simulink model "NewModuleTry_cs"  (Simulink 8.4)
settings: Solver=ode5  SolverMode=SingleTasking  StartTime=0.0  StopTime=inf  FixedStep=1/100  RelTol=1e-3
PreLoadFcn:
  | mbxruntime.callbacks.PreLoadFcn(bdroot);
PostLoadFcn:
  | mbxruntime.callbacks.PostLoadFcn(bdroot);
InitFcn:
  | mbxruntime.callbacks.InitFcn(bdroot);
StartFcn:
  | mbxruntime.callbacks.StartFcn(bdroot);
StopFcn:
  | mbxruntime.callbacks.StopFcn(bdroot);
undefined symbols (not defined in the file or in its folder): dfreq, gray, InitImageOutputDir, Rec, SDTV, strel
libraries: simulink x41, PreScanSimulinkLibrary x15, visiontextngfix x15, simulink_extras x12, visionconversions x3, PreScanUsefulBlocks x3, visionsinks x2, visionstatistics x1, visionmorphops x1, visionanalysis x1, simulink_need_slupdate x1
(part 2 of 7)

== system NewModuleTry_cs/BMW_Z3_1/DISABLED ==
  SELF_BMW_Z3_1 : Inport  Tag=inport/SelfPort  OutDataTypeStr=Bus: PRESCAN_SELFSENSORDATA  PortDimensions=1  SampleTime=1/100  BusOutputAsStruct=on
  TIS_1 : Inport  Tag=inport/TIS  Port=2  OutDataTypeStr=Bus: PRESCAN_SCANNERSENSOR_MESSAGE  PortDimensions=1  SampleTime=1/25  BusOutputAsStruct=on
  V2X_Rx243_Generic_Receiver : Inport  Tag=inport/plugin/sfun_V2X_Generic_Receiver  Port=3  BusOutputAsStruct=on
  GND1 : Subsystem
  GND2 : Ground
  TRM1 : Terminator
  TRM2 : Terminator
  TRM3 : Terminator
  STATE_BMW_Z3_1_bus : Outport  Tag=outport/StatePort  OutDataTypeStr=Bus: PRESCAN_STATEACTUATORDATA  PortDimensions=1  SampleTime=1/100
  V2X_Tx243_Generic_Transmitter : Outport  Tag=outport/plugin/sfun_V2X_Generic_Transmitter  Port=2
  wires:
  SELF_BMW_Z3_1/1 -> TRM1/1
  TIS_1/1 -> TRM2/1
  V2X_Rx243_Generic_Receiver/1 -> TRM3/1
  GND1/1(bus) -> STATE_BMW_Z3_1_bus/1
  GND2/1 -> V2X_Tx243_Generic_Transmitter/1

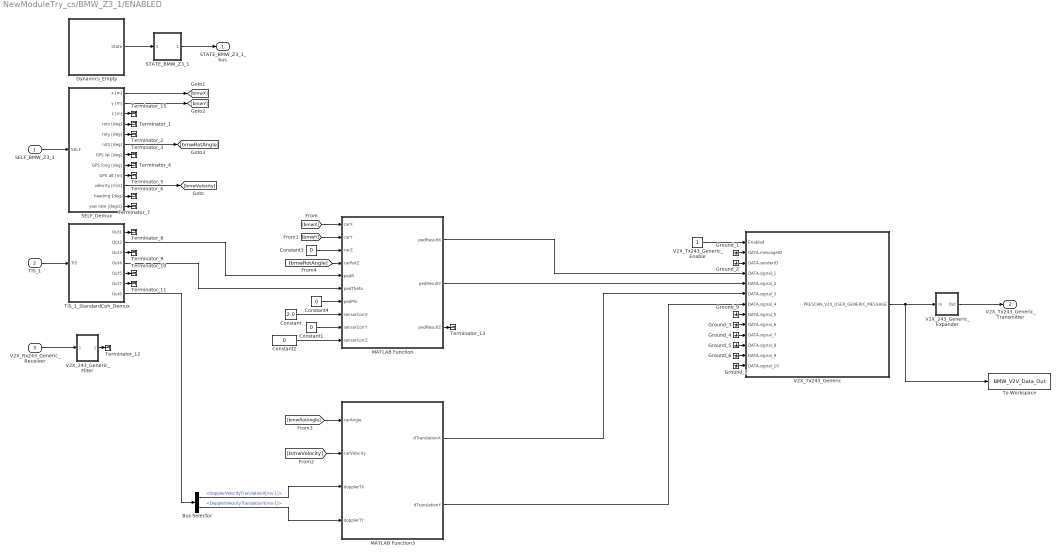
== system NewModuleTry_cs/BMW_Z3_1/ENABLED ==
  SELF_BMW_Z3_1 : Inport  Tag=inport/SelfPort  OutDataTypeStr=Bus: PRESCAN_SELFSENSORDATA  PortDimensions=1  SampleTime=1/100  BusOutputAsStruct=on
  TIS_1 : Inport  Tag=inport/TIS  Port=2  OutDataTypeStr=Bus: PRESCAN_SCANNERSENSOR_MESSAGE  PortDimensions=1  SampleTime=1/25  BusOutputAsStruct=on
  V2X_Rx243_Generic_Receiver : Inport  Tag=inport/plugin/sfun_V2X_Generic_Receiver  Port=3  BusOutputAsStruct=on
  Bus Selector : BusSelector  OutputSignals=DopplerVelocityTranslationX[ms-1],DopplerVelocityTranslationY[ms-1]
  Constant : Constant  Value=2.0
  Constant{1..4} (4 alike) : Constant  Value=0
  Dynamics_Empty : Subsystem  Tag=Dynamics_Empty
      mask Help: eval('openHelp(202)')
      mask Display: port_label('output', 1, 'State');text(0,0,' Empty\n')
  Ground_{1..7,9} (8 alike) : Ground
  MATLAB Function : MATLAB Function  TreatAsAtomicUnit=on
  MATLAB Function3 : MATLAB Function  TreatAsAtomicUnit=on
  SELF_Demux : Subsystem  Tag=demux/SelfPort  mask(PreScan Demux Block:){}
      mask help:
      | The SELF port shows (state) information of the actor itself. The outputs are position in the experiment's axis system and the GPS coordinates, and the object's absolute velocity and compass heading.
      |
      | For more information, please click Help.
      settings: DeleteFcn=PreScanBlockDeleteFcn;
      mask Help: eval('openHelp(462)')
      mask Display:
      | port_label('output',1,'x [m]')
      | port_label('output',2,'y [m]')
      | port_label('output',3,'z [m]','texmode','on')
      | port_label('output',4,'Rotx [deg]','texmode','on')
      | port_label('output',5,'Roty [deg]','texmode','on')
      | port_label('output',6,'Rotz [deg]','texmode','on')
      | port_label('output',7,'GPS lat [deg]','texmode','on')
      | port_label('output',8,'GPS long [deg]','texmode','on')
      | port_label('output',9,'GPS alt [m]','texmode','on')
      | port_label('output',10,'Velocity [m/s]')
      | port_label('output',11,'Heading [deg]')
      | port_label('output',12,'Yaw rate [deg/s]')
  STATE_BMW_Z3_1 : Subsystem  Tag=mux/StatePort  Priority=0  LoadFcn=load PrescanStateActuatorData  mask(PreScan Sink Block: State){x0=126.56578063964844, y0=141.80066680908203, z0=0.4784, Roll0=0, Pitch0=0, Yaw0=270, TimeStep=1/100}
      mask prompts: x0 "Ini x-position VEHICLE wrt GLOBAL axis system [m]"; y0 "Ini y-position VEHICLE wrt GLOBAL axis system [m]"; z0 "Ini z-position VEHICLE wrt GLOBAL axis system [m]"; Roll0 "Ini roll-angle BODY wrt VEHICLE axis system [deg]"; Pitch0 "Ini pitch-angle BODY wrt VEHICLE axis system [deg]"; Yaw0 "Ini yaw-angle VEHICLE wrt GLOBAL axis system [deg]"; TimeStep "Auto-Assigned: Upload Period [s]"
      mask help:
      | The Actor State contains a vector signal of size (9x1), containing the following signals:
      |
      | -  Position                  (x,y,z)                                     [m]
      | -  Velocity                  (vx,vy,vz)                               [m/s]
      | -  Angles                    (Roll, Pitch, Yaw)                   [rad]
      |
      | The Actor state is defined in the global axis system.
      | The state is superponed on the Initial position defined in the GUI.
      |
      | For more information, please click Help.
      settings: DeleteFcn=PreScanBlockDeleteFcn;
      mask Help: eval('openHelp(222)')
      mask Display: image(imread('State.png'))
  TIS_1_StandardCoh_Demux : Subsystem  Tag=demux/TIS/StandardCoh  TreatAsAtomicUnit=on  mask(PreScan Demux Block: TIS){MAXMESSAGES=1}
      mask prompts: MAXMESSAGES "Number of Objects"
      mask Help: eval('openHelp(449)')
      mask Display:
      | port_label('input',1,'TIS')
      | port_label('output',1,'Beam ID [-]')
      | port_label('output',2,'Range [m]')
      | port_label('output',3,'DopplerVelocity [m/s]')
      | port_label('output',4,'{\theta} [deg]','texmode','on')
      | port_label('output',5,'{\phi} [deg]','texmode','on')
      | port_label('output',6,'Target ID [-]','texmode','on')
      | port_label('output',7,'TIS Data','texmode','on')
  Terminator_{1..13,15} (14 alike) : Terminator
  To Workspace : ToWorkspace  VariableName=BMW_V2V_Data_Out  SaveFormat=Timeseries  SampleTime=-1
  V2X_243_Generic_Expander : Subsystem  LoadFcn=addpath .\V2XPlugin; V2Xbusses;
  V2X_243_Generic_Filter : Subsystem
      mask Display: disp('[1]');
  V2X_Tx243_Generic : Subsystem
  V2X_Tx243_Generic_Enable : Constant  OutDataTypeStr=Inherit: Inherit via back propagation
  STATE_BMW_Z3_1_bus : Outport  Tag=outport/StatePort  OutDataTypeStr=Bus: PRESCAN_STATEACTUATORDATA  PortDimensions=1  SampleTime=1/100
  V2X_Tx243_Generic_Transmitter : Outport  Tag=outport/plugin/sfun_V2X_Generic_Transmitter  Port=2
  wires:
  TIS_1_StandardCoh_Demux/2(Out2) -> MATLAB Function/5(pedR)
  TIS_1_StandardCoh_Demux/4(Out4) -> MATLAB Function/6(pedTheta)
  Constant/1 -> MATLAB Function/8(sensorCorrX)
  Constant1/1 -> MATLAB Function/9(sensorCorrY)
  Constant2/1 -> MATLAB Function/10(sensorCorrZ)
  Constant3/1 -> MATLAB Function/3(carZ)
  Constant4/1 -> MATLAB Function/7(pedPhi)
  SELF_Demux/3(z [m]) -> Terminator_15/1
  MATLAB Function/1(pedResultX) -> V2X_Tx243_Generic/4(DATA.signal_1)
  MATLAB Function/2(pedResultY) -> V2X_Tx243_Generic/5(DATA.signal_2)
  TIS_1_StandardCoh_Demux/7(Out6) -> Bus Selector/1
  Bus Selector/1 -> MATLAB Function3/3(dopplerTX)  "<DopplerVelocityTranslationX[ms-1]>"
  Bus Selector/2 -> MATLAB Function3/4(dopplerTY)  "<DopplerVelocityTranslationY[ms-1]>"
  SELF_Demux/10(velocity [m/s]) -> [bmwVelocity]
  SELF_Demux/1(x [m]) -> [bmwX]
  SELF_Demux/2(y [m]) -> [bmwY]
  [bmwX] -> MATLAB Function/1(carX)
  [bmwY] -> MATLAB Function/2(carY)
  SELF_Demux/6(rotz [deg]) -> [bmwRotAngle]
  [bmwVelocity] -> MATLAB Function3/2(carVelocity)
  [bmwRotAngle] -> MATLAB Function3/1(carAngle)
  MATLAB Function3/1(dTranslationX) -> V2X_Tx243_Generic/6(DATA.signal_3)
  MATLAB Function3/2(dTranslationY) -> V2X_Tx243_Generic/7(DATA.signal_4)
  [bmwRotAngle] -> MATLAB Function/4(carRotZ)
  Ground_9/1 -> V2X_Tx243_Generic/8(DATA.signal_5)
  MATLAB Function/3(pedResultZ) -> Terminator_13/1
  V2X_Tx243_Generic/1(PRESCAN_V2X_USER_GENERIC_MESSAGE) -> To Workspace/1, V2X_243_Generic_Expander/1(In)
  STATE_BMW_Z3_1/1(StateBus) -> STATE_BMW_Z3_1_bus/1
  SELF_BMW_Z3_1/1 -> SELF_Demux/1(SELF)
  TIS_1/1 -> TIS_1_StandardCoh_Demux/1(TIS)
  Dynamics_Empty/1(State) -> STATE_BMW_Z3_1/1(State)
  V2X_Tx243_Generic_Enable/1 -> V2X_Tx243_Generic/1(Enabled)
  V2X_243_Generic_Expander/1(Out) -> V2X_Tx243_Generic_Transmitter/1
  V2X_Rx243_Generic_Receiver/1 -> V2X_243_Generic_Filter/1(Filter_In)
  SELF_Demux/4(rotx [deg]) -> Terminator_1/1
  SELF_Demux/5(roty [deg]) -> Terminator_2/1
  SELF_Demux/7(GPS lat [deg]) -> Terminator_3/1
  SELF_Demux/8(GPS long [deg]) -> Terminator_4/1
  SELF_Demux/9(GPS alt [m]) -> Terminator_5/1
  SELF_Demux/11(heading [deg]) -> Terminator_6/1
  SELF_Demux/12(yaw rate [deg/s]) -> Terminator_7/1
  TIS_1_StandardCoh_Demux/1(Out1) -> Terminator_8/1
  TIS_1_StandardCoh_Demux/3(Out3) -> Terminator_9/1
  TIS_1_StandardCoh_Demux/5(Out5) -> Terminator_10/1
  TIS_1_StandardCoh_Demux/6(Out7) -> Terminator_11/1
  V2X_243_Generic_Filter/1(Filter_Out) -> Terminator_12/1
  Ground_1/1 -> V2X_Tx243_Generic/2(DATA.messageID)
  Ground_2/1 -> V2X_Tx243_Generic/3(DATA.senderID)
  Ground_3/1 -> V2X_Tx243_Generic/9(DATA.signal_6)
  Ground_4/1 -> V2X_Tx243_Generic/10(DATA.signal_7)
  Ground_5/1 -> V2X_Tx243_Generic/11(DATA.signal_8)
  Ground_6/1 -> V2X_Tx243_Generic/12(DATA.signal_9)
  Ground_7/1 -> V2X_Tx243_Generic/13(DATA.signal_10)

== system NewModuleTry_cs/CameraSensor_1/DISABLED ==
  GND1 : Ground
  CameraSensor_1 : Outport  Tag=outport/Camera/CameraSensor  OutDataTypeStr=uint8  SampleTime=1/50
  wires:
  GND1/1 -> CameraSensor_1/1

== system NewModuleTry_cs/CameraSensor_1/ENABLED ==
  Sensor : S-Function  FunctionName=sfun_Camera  Parameters=sensorID, dataWidth, dataHeight, channelsPerImage, numberOfImages, timestep  EnableBusSupport=off  mask(PreScan Source Block: Camera Sensor){sensorID=69, dataWidth=375, dataHeight=500, channelsPerImage=1, numberOfImages=1, timestep=1/50}
      mask prompts: sensorID "Sensor ID"; dataWidth "Data width"; dataHeight "Data Height"; channelsPerImage "Channels per image"; numberOfImages "Number of images"; timestep "MATLAB timestep:"
      mask help: The Camera Sensor provides a color or monochrome image.
      mask Help: eval('openHelp(457)')
      mask Display: image(imread('CameraSensor.png'))
  CameraSensor_1 : Outport  Tag=outport/Camera/CameraSensor  OutDataTypeStr=uint8  SampleTime=1/50
  wires:
  Sensor/1 -> CameraSensor_1/1

== system NewModuleTry_cs/CollisionDetection/DISABLED ==
  GND1 : Subsystem
  CollisionDetection : Outport  Tag=outport/CollisionDetection  OutDataTypeStr=Bus: PRESCAN_COLLISIONDETECTION_MESSAGE  PortDimensions=1  SampleTime=1/100
  wires:
  GND1/1(bus) -> CollisionDetection/1

== system NewModuleTry_cs/CollisionDetection/ENABLED ==
  Sensor : S-Function  FunctionName=sfun_CollisionDetection  Parameters=detectableCollisions, timestep  EnableBusSupport=off  mask(PreScan Source Block: CollisionDetection){detectableCollisions=1, timestep=1/100}
      mask prompts: detectableCollisions "Max detectable collisions:"; timestep "MATLAB timestep:"
      mask help: Collision Detection can be used to detect collisions between PreScan components. For Collision Detection the actual component shape is taken into account, so it is not a bounding box approach.
      mask Help: eval('openHelp(811)')
      mask Display: image(imread('crash.jpg'))
  CollisionDetection : Outport  Tag=outport/CollisionDetection  OutDataTypeStr=Bus: PRESCAN_COLLISIONDETECTION_MESSAGE  PortDimensions=1  SampleTime=1/100
  wires:
  Sensor/1 -> CollisionDetection/1

== system NewModuleTry_cs/Male_RegularAni_1/DISABLED ==
  SELF_Male_RegularAni_1 : Inport  Tag=inport/SelfPort  OutDataTypeStr=Bus: PRESCAN_SELFSENSORDATA  PortDimensions=1  SampleTime=1/100  BusOutputAsStruct=on
  GND1 : Subsystem
  GND2 : Subsystem
  TRM1 : Terminator
  STATE_Male_RegularAni_1_bus : Outport  Tag=outport/StatePort  OutDataTypeStr=Bus: PRESCAN_STATEACTUATORDATA  PortDimensions=1  SampleTime=1/100
  ANIM_Male_RegularAni_1 : Outport  Tag=outport/AnimationOutport  Port=2  OutDataTypeStr=Bus: PRESCAN_ANIMACTUATORDATA  PortDimensions=1  SampleTime=1/100
  wires:
  SELF_Male_RegularAni_1/1 -> TRM1/1
  GND1/1(bus) -> STATE_Male_RegularAni_1_bus/1
  GND2/1(bus) -> ANIM_Male_RegularAni_1/1

== system NewModuleTry_cs/Male_RegularAni_1/ENABLED ==
  SELF_Male_RegularAni_1 : Inport  Tag=inport/SelfPort  OutDataTypeStr=Bus: PRESCAN_SELFSENSORDATA  PortDimensions=1  SampleTime=1/100  BusOutputAsStruct=on
  Animation : Subsystem  Tag=RunningHumanAnimation  mask(Prescan Conversion Block: Running Human Animation){MWS=1.95, WalkingScale=1.0, RunningScale=1.0, TimeStep=1/100}
      mask prompts: MWS "Maximum Walking Speed [m/s], above which the animation will switch to running mode."; WalkingScale "Walking mode scaling factor to sync the animation frames to the displacement."; RunningScale "Running mode scaling factor to sync the animation frames to the displacement."; TimeStep "Auto-Assigned: Upload Period [s]"
      mask help: The Running Human Animation block converts the State signal of a human into signals to properly control the animation.
      mask Help: eval('openHelp(239)');
      mask Display: image(imread('HumanAnimated.jpg'))
  SELF_Demux : Subsystem  Tag=demux/SelfPort  mask(PreScan Demux Block:){}
      mask help:
      | The SELF port shows (state) information of the actor itself. The outputs are position in the experiment's axis system and the GPS coordinates, and the object's absolute velocity and compass heading.
      |
      | For more information, please click Help.
      settings: DeleteFcn=PreScanBlockDeleteFcn;
      mask Help: eval('openHelp(462)')
      mask Display:
      | port_label('output',1,'x [m]')
      | port_label('output',2,'y [m]')
      | port_label('output',3,'z [m]','texmode','on')
      | port_label('output',4,'Rotx [deg]','texmode','on')
      | port_label('output',5,'Roty [deg]','texmode','on')
      | port_label('output',6,'Rotz [deg]','texmode','on')
      | port_label('output',7,'GPS lat [deg]','texmode','on')
      | port_label('output',8,'GPS long [deg]','texmode','on')
      | port_label('output',9,'GPS alt [m]','texmode','on')
      | port_label('output',10,'Velocity [m/s]')
      | port_label('output',11,'Heading [deg]')
      | port_label('output',12,'Yaw rate [deg/s]')
  STATE_Male_RegularAni_1 : Subsystem  Tag=mux/StatePort  Priority=0  LoadFcn=load PrescanStateActuatorData  mask(PreScan Sink Block: State){x0=122.28665161132812, y0=124.52811431884766, z0=0, Roll0=0, Pitch0=0, Yaw0=53.000965224957312, TimeStep=1/100}
      mask prompts: x0 "Ini x-position VEHICLE wrt GLOBAL axis system [m]"; y0 "Ini y-position VEHICLE wrt GLOBAL axis system [m]"; z0 "Ini z-position VEHICLE wrt GLOBAL axis system [m]"; Roll0 "Ini roll-angle BODY wrt VEHICLE axis system [deg]"; Pitch0 "Ini pitch-angle BODY wrt VEHICLE axis system [deg]"; Yaw0 "Ini yaw-angle VEHICLE wrt GLOBAL axis system [deg]"; TimeStep "Auto-Assigned: Upload Period [s]"
      mask help:
      | The Actor State contains a vector signal of size (9x1), containing the following signals:
      |
      | -  Position                  (x,y,z)                                     [m]
      | -  Velocity                  (vx,vy,vz)                               [m/s]
      | -  Angles                    (Roll, Pitch, Yaw)                   [rad]
      |
      | The Actor state is defined in the global axis system.
      | The state is superponed on the Initial position defined in the GUI.
      |
      | For more information, please click Help.
      settings: DeleteFcn=PreScanBlockDeleteFcn;
      mask Help: eval('openHelp(222)')
      mask Display: image(imread('State.png'))
  Terminator_{1..12} (12 alike) : Terminator
  Trajectories : Subsystem  Tag=Trajectories  mask(PreScan Source Block: Trajectories){}
      mask help:
      | The Trajectory block contains the trajectories defined in the PreScan Experiment Editor. The output of the trajectory block is the (vehicle) State.
      |
      | For more information, please click Help.
      settings: DeleteFcn=PreScanBlockDeleteFcn;
      mask Help: eval('openHelp(312)')
      mask Display: image(imread('Trajectory.png'));
  STATE_Male_RegularAni_1_bus : Outport  Tag=outport/StatePort  OutDataTypeStr=Bus: PRESCAN_STATEACTUATORDATA  PortDimensions=1  SampleTime=1/100
  ANIM_Male_RegularAni_1 : Outport  Tag=outport/AnimationOutport  Port=2  OutDataTypeStr=Bus: PRESCAN_ANIMACTUATORDATA  PortDimensions=1  SampleTime=1/100
  wires:
  STATE_Male_RegularAni_1/1(StateBus) -> STATE_Male_RegularAni_1_bus/1, Animation/1(In1)
  Animation/1(Out1) -> ANIM_Male_RegularAni_1/1
  SELF_Male_RegularAni_1/1 -> SELF_Demux/1(SELF)
  Trajectories/1(State) -> STATE_Male_RegularAni_1/1(State)
  SELF_Demux/1(x [m]) -> Terminator_1/1
  SELF_Demux/2(y [m]) -> Terminator_2/1
  SELF_Demux/3(z [m]) -> Terminator_3/1
  SELF_Demux/4(rotx [deg]) -> Terminator_4/1
  SELF_Demux/5(roty [deg]) -> Terminator_5/1
  SELF_Demux/6(rotz [deg]) -> Terminator_6/1
  SELF_Demux/7(GPS lat [deg]) -> Terminator_7/1
  SELF_Demux/8(GPS long [deg]) -> Terminator_8/1
  SELF_Demux/9(GPS alt [m]) -> Terminator_9/1
  SELF_Demux/10(velocity [m/s]) -> Terminator_10/1
  SELF_Demux/11(heading [deg]) -> Terminator_11/1
  SELF_Demux/12(yaw rate [deg/s]) -> Terminator_12/1

== system NewModuleTry_cs/SELF_Audi_A8_1/DISABLED ==
  GND1 : Subsystem
  SELF_Audi_A8_1 : Outport  Tag=outport/SelfPort  OutDataTypeStr=Bus: PRESCAN_SELFSENSORDATA  PortDimensions=1  SampleTime=1/100
  wires:
  GND1/1(bus) -> SELF_Audi_A8_1/1

== system NewModuleTry_cs/SELF_Audi_A8_1/ENABLED ==
  Sensor : S-Function  FunctionName=sfun_SelfSensor  Parameters=UniqueID, TimeStep  EnableBusSupport=off  mask(PreScan Source Block: SELF){UniqueID=58, TimeStep=1/100}
      mask prompts: UniqueID "Auto-Assigned: Unique ID"; TimeStep "Auto-Assigned: Upload Period [s]"
      mask help:
      | The SELF port shows (state) information of the actor itself. The outputs are position in the experiment's axis system and the GPS coordinates, and the object's absolute velocity and compass heading.
      |
      | For more information, please click Help.
      mask Help: eval('openHelp(462)')
      mask Display: image(imread('GPS.png'))
  SELF_Audi_A8_1 : Outport  Tag=outport/SelfPort  OutDataTypeStr=Bus: PRESCAN_SELFSENSORDATA  PortDimensions=1  SampleTime=1/100
  wires:
  Sensor/1 -> SELF_Audi_A8_1/1

== system NewModuleTry_cs/SELF_BMW_Z3_1/DISABLED ==
  GND1 : Subsystem
  SELF_BMW_Z3_1 : Outport  Tag=outport/SelfPort  OutDataTypeStr=Bus: PRESCAN_SELFSENSORDATA  PortDimensions=1  SampleTime=1/100
  wires:
  GND1/1(bus) -> SELF_BMW_Z3_1/1

== system NewModuleTry_cs/SELF_BMW_Z3_1/ENABLED ==
  Sensor : S-Function  FunctionName=sfun_SelfSensor  Parameters=UniqueID, TimeStep  EnableBusSupport=off  mask(PreScan Source Block: SELF){UniqueID=59, TimeStep=1/100}
      mask prompts: UniqueID "Auto-Assigned: Unique ID"; TimeStep "Auto-Assigned: Upload Period [s]"
      mask help:
      | The SELF port shows (state) information of the actor itself. The outputs are position in the experiment's axis system and the GPS coordinates, and the object's absolute velocity and compass heading.
      |
      | For more information, please click Help.
      mask Help: eval('openHelp(462)')
      mask Display: image(imread('GPS.png'))
  SELF_BMW_Z3_1 : Outport  Tag=outport/SelfPort  OutDataTypeStr=Bus: PRESCAN_SELFSENSORDATA  PortDimensions=1  SampleTime=1/100
  wires:
  Sensor/1 -> SELF_BMW_Z3_1/1

== system NewModuleTry_cs/SELF_Male_RegularAni_1/DISABLED ==
  GND1 : Subsystem
  SELF_Male_RegularAni_1 : Outport  Tag=outport/SelfPort  OutDataTypeStr=Bus: PRESCAN_SELFSENSORDATA  PortDimensions=1  SampleTime=1/100
  wires:
  GND1/1(bus) -> SELF_Male_RegularAni_1/1

== system NewModuleTry_cs/SELF_Male_RegularAni_1/ENABLED ==
  Sensor : S-Function  FunctionName=sfun_SelfSensor  Parameters=UniqueID, TimeStep  EnableBusSupport=off  mask(PreScan Source Block: SELF){UniqueID=60, TimeStep=1/100}
      mask prompts: UniqueID "Auto-Assigned: Unique ID"; TimeStep "Auto-Assigned: Upload Period [s]"
      mask help:
      | The SELF port shows (state) information of the actor itself. The outputs are position in the experiment's axis system and the GPS coordinates, and the object's absolute velocity and compass heading.
      |
      | For more information, please click Help.
      mask Help: eval('openHelp(462)')
      mask Display: image(imread('GPS.png'))
  SELF_Male_RegularAni_1 : Outport  Tag=outport/SelfPort  OutDataTypeStr=Bus: PRESCAN_SELFSENSORDATA  PortDimensions=1  SampleTime=1/100
  wires:
  Sensor/1 -> SELF_Male_RegularAni_1/1

== system NewModuleTry_cs/STATE_Audi_A8_1_bus/DISABLED ==
  STATE_Audi_A8_1_bus : Inport  Tag=inport/StatePort  OutDataTypeStr=Bus: PRESCAN_STATEACTUATORDATA  PortDimensions=1  SampleTime=1/100  BusOutputAsStruct=on
  TRM1 : Terminator
  wires:
  STATE_Audi_A8_1_bus/1 -> TRM1/1

== system NewModuleTry_cs/STATE_Audi_A8_1_bus/ENABLED ==
  STATE_Audi_A8_1_bus : Inport  Tag=inport/StatePort  OutDataTypeStr=Bus: PRESCAN_STATEACTUATORDATA  PortDimensions=1  SampleTime=1/100  BusOutputAsStruct=on
  Actuator : S-Function  FunctionName=sfun_StateActuator  Parameters=UniqueID, TimeStep  EnableBusSupport=off  mask(PreScan Sink Block: State){UniqueID=58, TimeStep=1/100}
      mask prompts: UniqueID "Auto-Assigned: Unique ID"; TimeStep "Auto-Assigned: Upload Period [s]"
      mask help:
      | The Actor State contains a vector signal of size (9x1), containing the following signals:
      |
      | -  Position    	(x,y,z)             	[m]
      | -  Velocity    	(vx,vy,vz)         	[m/s]
      | -  Angles       	(Roll, Pitch, Yaw)	[rad]
      |
      | The Actor state is defined in the global axis system.
      | The state is superponed on the Initial position defined in the GUI.
      |
      | For more information, please click Help.
      mask Help: eval('openHelp(222)')
      mask Display: image(imread('State.png'))
  wires:
  STATE_Audi_A8_1_bus/1 -> Actuator/1

== system NewModuleTry_cs/STATE_BMW_Z3_1_bus/DISABLED ==
  STATE_BMW_Z3_1_bus : Inport  Tag=inport/StatePort  OutDataTypeStr=Bus: PRESCAN_STATEACTUATORDATA  PortDimensions=1  SampleTime=1/100  BusOutputAsStruct=on
  TRM1 : Terminator
  wires:
  STATE_BMW_Z3_1_bus/1 -> TRM1/1

== system NewModuleTry_cs/STATE_BMW_Z3_1_bus/ENABLED ==
  STATE_BMW_Z3_1_bus : Inport  Tag=inport/StatePort  OutDataTypeStr=Bus: PRESCAN_STATEACTUATORDATA  PortDimensions=1  SampleTime=1/100  BusOutputAsStruct=on
  Actuator : S-Function  FunctionName=sfun_StateActuator  Parameters=UniqueID, TimeStep  EnableBusSupport=off  mask(PreScan Sink Block: State){UniqueID=59, TimeStep=1/100}
      mask prompts: UniqueID "Auto-Assigned: Unique ID"; TimeStep "Auto-Assigned: Upload Period [s]"
      mask help:
      | The Actor State contains a vector signal of size (9x1), containing the following signals:
      |
      | -  Position    	(x,y,z)             	[m]
      | -  Velocity    	(vx,vy,vz)         	[m/s]
      | -  Angles       	(Roll, Pitch, Yaw)	[rad]
      |
      | The Actor state is defined in the global axis system.
      | The state is superponed on the Initial position defined in the GUI.
      |
      | For more information, please click Help.
      mask Help: eval('openHelp(222)')
      mask Display: image(imread('State.png'))
  wires:
  STATE_BMW_Z3_1_bus/1 -> Actuator/1

== system NewModuleTry_cs/STATE_Male_RegularAni_1_bus/DISABLED ==
  STATE_Male_RegularAni_1_bus : Inport  Tag=inport/StatePort  OutDataTypeStr=Bus: PRESCAN_STATEACTUATORDATA  PortDimensions=1  SampleTime=1/100  BusOutputAsStruct=on
  TRM1 : Terminator
  wires:
  STATE_Male_RegularAni_1_bus/1 -> TRM1/1

== system NewModuleTry_cs/STATE_Male_RegularAni_1_bus/ENABLED ==
  STATE_Male_RegularAni_1_bus : Inport  Tag=inport/StatePort  OutDataTypeStr=Bus: PRESCAN_STATEACTUATORDATA  PortDimensions=1  SampleTime=1/100  BusOutputAsStruct=on
  Actuator : S-Function  FunctionName=sfun_StateActuator  Parameters=UniqueID, TimeStep  EnableBusSupport=off  mask(PreScan Sink Block: State){UniqueID=60, TimeStep=1/100}
      mask prompts: UniqueID "Auto-Assigned: Unique ID"; TimeStep "Auto-Assigned: Upload Period [s]"
      mask help:
      | The Actor State contains a vector signal of size (9x1), containing the following signals:
      |
      | -  Position    	(x,y,z)             	[m]
      | -  Velocity    	(vx,vy,vz)         	[m/s]
      | -  Angles       	(Roll, Pitch, Yaw)	[rad]
      |
      | The Actor state is defined in the global axis system.
      | The state is superponed on the Initial position defined in the GUI.
      |
      | For more information, please click Help.
      mask Help: eval('openHelp(222)')
      mask Display: image(imread('State.png'))
  wires:
  STATE_Male_RegularAni_1_bus/1 -> Actuator/1

== system NewModuleTry_cs/TIS_1/DISABLED ==
  GND1 : Subsystem
  TIS_1 : Outport  Tag=outport/TIS  OutDataTypeStr=Bus: PRESCAN_SCANNERSENSOR_MESSAGE  PortDimensions=1  SampleTime=1/25
  wires:
  GND1/1(bus) -> TIS_1/1

== system NewModuleTry_cs/TIS_1/ENABLED ==
  Sensor : S-Function  FunctionName=sfun_TIS  Parameters=sensorID, detectableObjects, timestep  EnableBusSupport=off  mask(PreScan Source Block: Technology Independent Sensor (TIS)){sensorID=68, detectableObjects=1, timestep=1/25}
      mask prompts: sensorID "Sensor ID"; detectableObjects "Max detectable objects:"; timestep "MATLAB timestep:"
      mask help:
      | The Technology Independent Sensor (TIS) provides a sensor with all sensor-related influence factors (like noise, drift and accuracy) without being technology specific (like radar and lidar). The TIS detects the closest point on the geometry of an object.
      |
      | For more information, please click Help.
      mask Help: eval('openHelp(449)')
      mask Display: image(imread('TIS.png'))
  TIS_1 : Outport  Tag=outport/TIS  OutDataTypeStr=Bus: PRESCAN_SCANNERSENSOR_MESSAGE  PortDimensions=1  SampleTime=1/25
  wires:
  Sensor/1 -> TIS_1/1

== system NewModuleTry_cs/TIS_2/DISABLED ==
  GND1 : Subsystem
  TIS_2 : Outport  Tag=outport/TIS  OutDataTypeStr=Bus: PRESCAN_SCANNERSENSOR_MESSAGE  PortDimensions=1  SampleTime=1/25
  wires:
  GND1/1(bus) -> TIS_2/1

== system NewModuleTry_cs/TIS_2/ENABLED ==
  Sensor : S-Function  FunctionName=sfun_TIS  Parameters=sensorID, detectableObjects, timestep  EnableBusSupport=off  mask(PreScan Source Block: Technology Independent Sensor (TIS)){sensorID=192, detectableObjects=1, timestep=1/25}
      mask prompts: sensorID "Sensor ID"; detectableObjects "Max detectable objects:"; timestep "MATLAB timestep:"
      mask help:
      | The Technology Independent Sensor (TIS) provides a sensor with all sensor-related influence factors (like noise, drift and accuracy) without being technology specific (like radar and lidar). The TIS detects the closest point on the geometry of an object.
      |
      | For more information, please click Help.
      mask Help: eval('openHelp(449)')
      mask Display: image(imread('TIS.png'))
  TIS_2 : Outport  Tag=outport/TIS  OutDataTypeStr=Bus: PRESCAN_SCANNERSENSOR_MESSAGE  PortDimensions=1  SampleTime=1/25
  wires:
  Sensor/1 -> TIS_2/1

== system NewModuleTry_cs/V2X_Rx243_Generic_Receiver/DISABLED ==
  GND1 : Ground
  V2X_Rx243_Generic_Receiver : Outport  Tag=outport/plugin/sfun_V2X_Generic_Receiver
  wires:
  GND1/1 -> V2X_Rx243_Generic_Receiver/1

== system NewModuleTry_cs/V2X_Rx243_Generic_Receiver/ENABLED ==
  Sensor : S-Function  LoadFcn=load('Generic.mat');  FunctionName=sfun_V2X_Generic_Receiver  Parameters=sensorID, parentID, maxMessages, timestep  EnableBusSupport=off  mask(V2X Generic Receiver Block){sensorID=243, parentID=59, maxMessages=1, timestep=1/100}
      mask prompts: sensorID "Receiver ID"; parentID "Parent ID"; maxMessages "Maximum number of messages"; timestep "MATLAB timestep:"
      mask help: V2X Block receiving a Generic message
      mask Display: image(imread('V2XR_grayscale.png'))
  V2X_Rx243_Generic_Receiver : Outport  Tag=outport/plugin/sfun_V2X_Generic_Receiver
  wires:
  Sensor/1 -> V2X_Rx243_Generic_Receiver/1

== system NewModuleTry_cs/V2X_Rx244_Generic_Receiver/DISABLED ==
  GND1 : Ground
  V2X_Rx244_Generic_Receiver : Outport  Tag=outport/plugin/sfun_V2X_Generic_Receiver
  wires:
  GND1/1 -> V2X_Rx244_Generic_Receiver/1

== system NewModuleTry_cs/V2X_Rx244_Generic_Receiver/ENABLED ==
  Sensor : S-Function  LoadFcn=load('Generic.mat');  FunctionName=sfun_V2X_Generic_Receiver  Parameters=sensorID, parentID, maxMessages, timestep  EnableBusSupport=off  mask(V2X Generic Receiver Block){sensorID=244, parentID=58, maxMessages=1, timestep=1/100}
      mask prompts: sensorID "Receiver ID"; parentID "Parent ID"; maxMessages "Maximum number of messages"; timestep "MATLAB timestep:"
      mask help: V2X Block receiving a Generic message
      mask Display: image(imread('V2XR_grayscale.png'))
  V2X_Rx244_Generic_Receiver : Outport  Tag=outport/plugin/sfun_V2X_Generic_Receiver
  wires:
  Sensor/1 -> V2X_Rx244_Generic_Receiver/1

== system NewModuleTry_cs/V2X_Tx243_Generic_Transmitter/DISABLED ==
  V2X_Tx243_Generic_Transmitter : Inport  Tag=inport/plugin/sfun_V2X_Generic_Transmitter  BusOutputAsStruct=on
  TRM1 : Terminator
  wires:
  V2X_Tx243_Generic_Transmitter/1 -> TRM1/1

== system NewModuleTry_cs/V2X_Tx243_Generic_Transmitter/ENABLED ==
  V2X_Tx243_Generic_Transmitter : Inport  Tag=inport/plugin/sfun_V2X_Generic_Transmitter  BusOutputAsStruct=on
  Actuator : S-Function  LoadFcn=load('Generic.mat');  FunctionName=sfun_V2X_Generic_Transmitter  Parameters=sensorID, parentID, timestep  EnableBusSupport=off  mask(V2X Generic Transmitter Block){sensorID=243, parentID=59, timestep=1/100}
      mask prompts: sensorID "Transmitter ID"; parentID "Parent ID"; timestep "MATLAB timestep:"
      mask help: V2X Block transmitting a Generic message
      mask Display: image(imread('V2XT_grayscale.png'))
  wires:
  V2X_Tx243_Generic_Transmitter/1 -> Actuator/1

== system NewModuleTry_cs/V2X_Tx244_Generic_Transmitter/DISABLED ==
  V2X_Tx244_Generic_Transmitter : Inport  Tag=inport/plugin/sfun_V2X_Generic_Transmitter  BusOutputAsStruct=on
  TRM1 : Terminator
  wires:
  V2X_Tx244_Generic_Transmitter/1 -> TRM1/1

== system NewModuleTry_cs/V2X_Tx244_Generic_Transmitter/ENABLED ==
  V2X_Tx244_Generic_Transmitter : Inport  Tag=inport/plugin/sfun_V2X_Generic_Transmitter  BusOutputAsStruct=on
  Actuator : S-Function  LoadFcn=load('Generic.mat');  FunctionName=sfun_V2X_Generic_Transmitter  Parameters=sensorID, parentID, timestep  EnableBusSupport=off  mask(V2X Generic Transmitter Block){sensorID=244, parentID=58, timestep=1/100}
      mask prompts: sensorID "Transmitter ID"; parentID "Parent ID"; timestep "MATLAB timestep:"
      mask help: V2X Block transmitting a Generic message
      mask Display: image(imread('V2XT_grayscale.png'))
  wires:
  V2X_Tx244_Generic_Transmitter/1 -> Actuator/1

== system NewModuleTry_cs/Audi_A8_1/DISABLED/GND1 ==
  GND_AccelerationX : Constant  Value=0
  GND_AccelerationY : Constant  Value=0
  GND_AccelerationZ : Constant  Value=0
  GND_AngularVelocityPitch : Constant  Value=0
  GND_AngularVelocityRoll : Constant  Value=0
  GND_AngularVelocityYaw : Constant  Value=0
  GND_OrientationPitch : Constant  Value=0
  GND_OrientationRoll : Constant  Value=0
  GND_OrientationYaw : Constant  Value=0
  GND_PositionX : Constant  Value=0
  GND_PositionY : Constant  Value=0
  GND_PositionZ : Constant  Value=0
  GND_VelocityX : Constant  Value=0
  GND_VelocityY : Constant  Value=0
  GND_VelocityZ : Constant  Value=0
  buscreator : BusCreator  Inputs=15  OutDataTypeStr=Bus: PRESCAN_STATEACTUATORDATA  NonVirtualBus=on
  bus : Outport  OutDataTypeStr=Bus: PRESCAN_STATEACTUATORDATA
  wires:
  GND_PositionX/1 -> buscreator/1  "PositionX"
  GND_PositionY/1 -> buscreator/2  "PositionY"
  GND_PositionZ/1 -> buscreator/3  "PositionZ"
  GND_VelocityX/1 -> buscreator/4  "VelocityX"
  GND_VelocityY/1 -> buscreator/5  "VelocityY"
  GND_VelocityZ/1 -> buscreator/6  "VelocityZ"
  GND_AccelerationX/1 -> buscreator/7  "AccelerationX"
  GND_AccelerationY/1 -> buscreator/8  "AccelerationY"
  GND_AccelerationZ/1 -> buscreator/9  "AccelerationZ"
  GND_OrientationRoll/1 -> buscreator/10  "OrientationRoll"
  GND_OrientationPitch/1 -> buscreator/11  "OrientationPitch"
  GND_OrientationYaw/1 -> buscreator/12  "OrientationYaw"
  GND_AngularVelocityRoll/1 -> buscreator/13  "AngularVelocityRoll"
  GND_AngularVelocityPitch/1 -> buscreator/14  "AngularVelocityPitch"
  GND_AngularVelocityYaw/1 -> buscreator/15  "AngularVelocityYaw"
  buscreator/1 -> bus/1

== system NewModuleTry_cs/Audi_A8_1/ENABLED/CameraSensor_1_MM_Demux ==
  note: This block exists for legacy compatibility only
  In1 : Inport
  I : Outport
  wires:
  In1/1 -> I/1

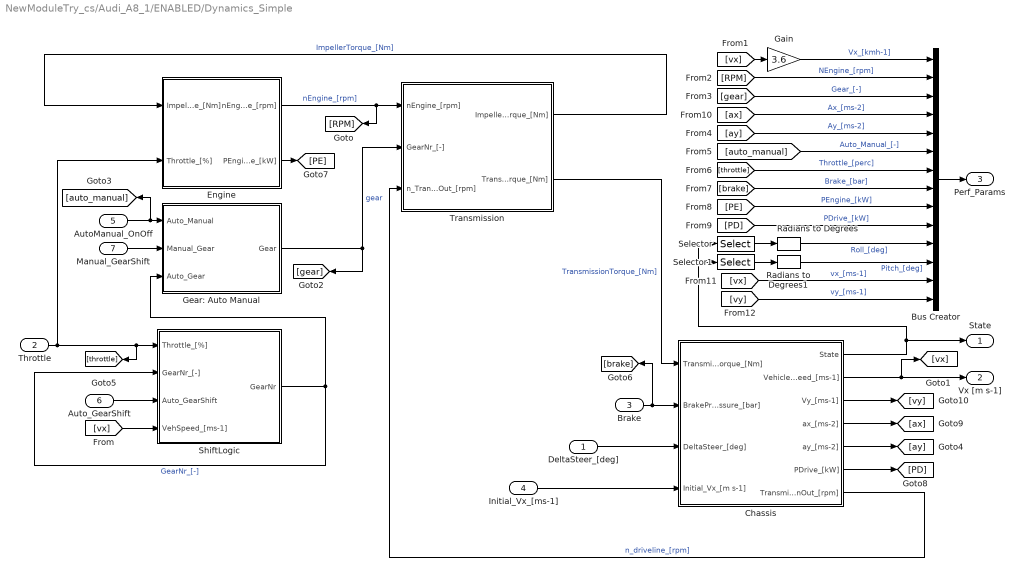
== system NewModuleTry_cs/Audi_A8_1/ENABLED/Dynamics_Simple ==
  DeltaSteer_[deg] : Inport
  Throttle : Inport  Port=2
  Brake : Inport  Port=3
  Initial_Vx_[ms-1] : Inport  Port=4
  AutoManual_OnOff : Inport  Port=5
  Auto_GearShift : Inport  Port=6
  Manual_GearShift : Inport  Port=7
  Bus Creator : BusCreator  Inputs=14
  Chassis : Subsystem
      mask Display: image(imread('Chassis.png'));
  Engine : Subsystem
      mask Display: image(imread('Engine.png'));
  Gain : Gain  Gain=3.6
  Gear: Auto Manual : Subsystem
  Radians to Degrees : simulink_extras/Transformations/Radians to Degrees
  Radians to Degrees1 : simulink_extras/Transformations/Radians to Degrees
  Selector : Selector  InputPortWidth=9  Indices=7
  Selector1 : Selector  InputPortWidth=9  Indices=8
  ShiftLogic : Subsystem
      mask Display: image(imread('Gearshift.png'));
  Transmission : Subsystem
      mask Display: image(imread('Transmission.png'));
  State : Outport
  Vx [m s-1] : Outport  Port=2
  Perf_Params : Outport  Port=3
  wires:
  [vy] -> Bus Creator/14  "vy_[ms-1]"
  [vx] -> Bus Creator/13  "vx_[ms-1]"
  Chassis/7(TransmissionOut_[rpm]) -> Transmission/3(n_TransmissionOut_[rpm])  "n_driveline_[rpm]"
  Chassis/6(PDrive_[kW]) -> [PD]
  Chassis/5(ay_[ms-2]) -> [ay]
  Chassis/4(ax_[ms-2]) -> [ax]
  Chassis/3(Vy_[ms-1]) -> [vy]
  [vx] -> ShiftLogic/4(VehSpeed_[ms-1])
  Gear: Auto Manual/1(Gear) -> Transmission/2(GearNr_[-]), [gear]  "gear"
  Manual_GearShift/1 -> Gear: Auto Manual/2(Manual_Gear)
  AutoManual_OnOff/1 -> Gear: Auto Manual/1(Auto_Manual), [auto_manual]
  Chassis/2(VehicleSpeed_[ms-1]) -> [vx], Vx [m s-1]/1
  Auto_GearShift/1 -> ShiftLogic/3(Auto_GearShift)
  Throttle/1 -> Engine/2(Throttle_[%]), ShiftLogic/1(Throttle_[%]), [throttle]
  Initial_Vx_[ms-1]/1 -> Chassis/4(Initial_Vx_[m s-1])
  DeltaSteer_[deg]/1 -> Chassis/3(DeltaSteer_[deg])
  Chassis/1(State) -> State/1, Selector/1, Selector1/1
  Brake/1 -> [brake], Chassis/2(BrakePressure_[bar])
  Engine/1(nEngine_[rpm]) -> [RPM], Transmission/1(nEngine_[rpm])  "nEngine_[rpm]"
  ShiftLogic/1(GearNr) -> Gear: Auto Manual/3(Auto_Gear), ShiftLogic/2(GearNr_[-])  "GearNr_[-]"
  Transmission/2(TransmissionTorque_[Nm]) -> Chassis/1(TransmissionTorque_[Nm])  "TransmissionTorque_[Nm]"
  Transmission/1(ImpellerTorque_[Nm]) -> Engine/1(ImpellerTorque_[Nm])  "ImpellerTorque_[Nm]"
  Gain/1 -> Bus Creator/1  "Vx_[kmh-1]"
  [RPM] -> Bus Creator/2  "NEngine_[rpm]"
  [gear] -> Bus Creator/3  "Gear_[-]"
  [ay] -> Bus Creator/5  "Ay_[ms-2]"
  [auto_manual] -> Bus Creator/6  "Auto_Manual_[-]"
  [throttle] -> Bus Creator/7  "Throttle_[perc]"
  [brake] -> Bus Creator/8  "Brake_[bar]"
  Engine/2(PEngine_[kW]) -> [PE]
  Bus Creator/1 -> Perf_Params/1
  [PE] -> Bus Creator/9  "PEngine_[kW]"
  Radians to Degrees/1 -> Bus Creator/11  "Roll_[deg]"
  Radians to Degrees1/1 -> Bus Creator/12  "Pitch_[deg]"
  [PD] -> Bus Creator/10  "PDrive_[kW]"
  Selector/1 -> Radians to Degrees/1
  Selector1/1 -> Radians to Degrees1/1
  [vx] -> Gain/1
  [ax] -> Bus Creator/4  "Ax_[ms-2]"

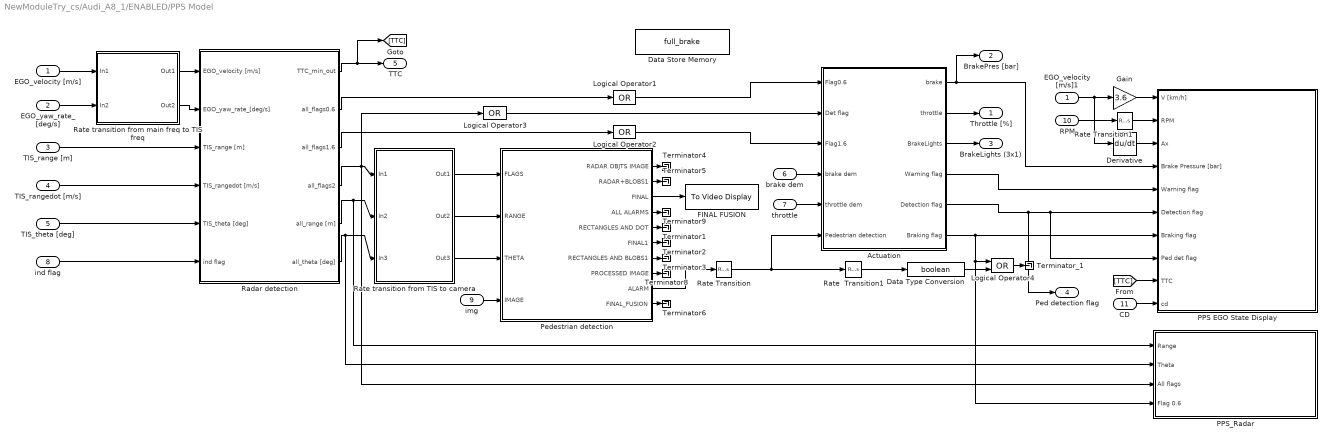
== system NewModuleTry_cs/Audi_A8_1/ENABLED/PPS Model ==
  EGO_velocity [m/s] : Inport
  EGO_yaw_rate_[deg/s] : Inport  Port=2  SampleTime=1/Mainfreq
  TIS_range [m] : Inport  Port=3  PortDimensions=TISdet  SampleTime=1/TISfreq
  TIS_rangedot [m/s] : Inport  Port=4  PortDimensions=TISdet  SampleTime=1/TISfreq
  TIS_theta [deg] : Inport  Port=5  PortDimensions=TISdet  SampleTime=1/TISfreq
  brake dem : Inport  Port=6  SampleTime=[0,0]
  throttle : Inport  Port=7  SampleTime=[0,0]
  ind flag : Inport  Port=8  SampleTime=1/TISfreq
  img : Inport  Port=9  PortDimensions=[375 500]  SampleTime=1/Camfreq
  RPM : Inport  Port=10
  CD : Inport  Port=11
  Actuation : Subsystem
  Data Store Memory : DataStoreMemory  DataStoreName=full_brake  ReadBeforeWriteMsg=warning  WriteAfterWriteMsg=warning  WriteAfterReadMsg=warning
  Data Type Conversion : DataTypeConversion  OutDataTypeStr=boolean
  Derivative : Derivative
  EGO_velocity [m/s]1 : InportShadow
  FINAL FUSION : visionsinks/To Video Display  inputType=Obsolete  imagePorts=One multidimensional signal  OutputDevice=On-screen video monitor  fullScreen=off  videoWindowX=1279  videoWindowY=19  saveWindowSize=off  videoWindowWidth=500  videoWindowHeight=375  dataOrg=Column-major  openAtMdlStart=on  isWindowOpen=off  inputColorFormat=RGB
  Gain : Gain  Gain=3.6
  Logical Operator1 : Logic  Operator=OR  Inputs=1  AllPortsSameDT=off  OutDataTypeStr=boolean
  Logical Operator2 : Logic  Operator=OR  Inputs=1  AllPortsSameDT=off  OutDataTypeStr=boolean
  Logical Operator3 : Logic  Operator=OR  Inputs=1  AllPortsSameDT=off  OutDataTypeStr=boolean
  Logical Operator4 : Logic  Operator=OR  AllPortsSameDT=off  OutDataTypeStr=boolean
  PPS EGO State Display : Subsystem
  PPS_Radar : Subsystem
  Pedestrian detection : Subsystem
  Radar detection : Subsystem
  Rate  Transition1 : RateTransition  Integrity=off  Deterministic=off  OutPortSampleTime=1/min(TISfreq,Camfreq)
  Rate Transition : RateTransition  Integrity=off  Deterministic=off  OutPortSampleTime=[0,0]
  Rate Transition1 : RateTransition  Integrity=off  Deterministic=off  OutPortSampleTime=1/Mainfreq
  Rate transition from TIS to camera : Subsystem
  Rate transition from main freq to TIS freq : Subsystem
  Terminator{1..6,8..9} (8 alike) : Terminator
  Terminator_1 : Terminator
  Throttle [%] : Outport
  BrakePres [bar] : Outport  Port=2
  BrakeLights (3x1) : Outport  Port=3
  Ped detection flag : Outport  Port=4  PortDimensions=1
  TTC : Outport  Port=5
  wires:
  TIS_range [m]/1 -> Radar detection/3(TIS_range [m])
  TIS_rangedot [m/s]/1 -> Radar detection/4(TIS_rangedot [m/s])
  TIS_theta [deg]/1 -> Radar detection/5(TIS_theta [deg])
  ind flag/1 -> Radar detection/6(ind flag)
  EGO_velocity [m/s]/1 -> Rate transition from main freq to TIS freq/1(In1)
  EGO_yaw_rate_[deg/s]/1 -> Rate transition from main freq to TIS freq/2(In2)
  Rate transition from main freq to TIS freq/1(Out1) -> Radar detection/1(EGO_velocity [m/s])
  Rate transition from main freq to TIS freq/2(Out2) -> Radar detection/2(EGO_yaw_rate_[deg/s])
  throttle/1 -> Actuation/5(throttle dem)
  brake dem/1 -> Actuation/4(brake dem)
  Radar detection/1(TTC_min_out) -> TTC/1, [TTC]
  Radar detection/2(all_flags0.6) -> Logical Operator1/1
  Rate Transition/1 -> Actuation/6(Pedestrian detection), Rate  Transition1/1
  Rate  Transition1/1 -> Data Type Conversion/1
  Radar detection/4(all_flags2) -> Rate transition from TIS to camera/1(In1), Logical Operator3/1, PPS_Radar/3(All flags)
  Radar detection/5(all_range [m]) -> Rate transition from TIS to camera/2(In2), PPS_Radar/1(Range)
  Radar detection/6(all_theta [deg]) -> Rate transition from TIS to camera/3(In3), PPS_Radar/2(Theta)
  Radar detection/3(all_flags1.6) -> Logical Operator2/1
  Actuation/1(brake) -> BrakePres [bar]/1, PPS EGO State Display/4(Brake Pressure [bar])
  Actuation/2(throttle) -> Throttle [%]/1
  Actuation/3(BrakeLights) -> BrakeLights (3x1)/1
  Actuation/6(Braking flag) -> PPS EGO State Display/7(Braking flag), Logical Operator4/1, PPS_Radar/4(Flag 0.6)
  Pedestrian detection/8(PROCESSED IMAGE) -> Terminator8/1
  Pedestrian detection/4(ALL ALARMS) -> Terminator9/1
  Pedestrian detection/5(RECTANGLES AND DOT) -> Terminator1/1
  Pedestrian detection/7(RECTANGLES AND BLOBS1) -> Terminator3/1
  Pedestrian detection/2(RADAR+BLOBS1) -> Terminator5/1
  Pedestrian detection/1(RADAR OBJTS IMAGE) -> Terminator4/1
  Pedestrian detection/10(FINAL_FUSION) -> Terminator6/1
  img/1 -> Pedestrian detection/4(IMAGE)
  Pedestrian detection/3(FINAL) -> FINAL FUSION/1
  Pedestrian detection/6(FINAL1) -> Terminator2/1
  Rate transition from TIS to camera/1(Out1) -> Pedestrian detection/1(FLAGS)
  Rate transition from TIS to camera/2(Out2) -> Pedestrian detection/2(RANGE)
  Rate transition from TIS to camera/3(Out3) -> Pedestrian detection/3(THETA)
  Logical Operator1/1 -> Actuation/1(Flag0.6)
  Logical Operator2/1 -> Actuation/3(Flag1.6)
  Logical Operator3/1 -> Actuation/2(Det flag)
  EGO_velocity [m/s]1/1 -> Gain/1, Derivative/1
  Gain/1 -> PPS EGO State Display/1(V [km/h])
  RPM/1 -> Rate Transition1/1
  Derivative/1 -> PPS EGO State Display/3(Ax)
  CD/1 -> PPS EGO State Display/10(cd)
  [TTC] -> PPS EGO State Display/9(TTC)
  Actuation/4(Warning flag) -> PPS EGO State Display/5(Warning flag)
  Actuation/5(Detection flag) -> Ped detection flag/1, PPS EGO State Display/8(Ped det flag), PPS EGO State Display/6(Detection flag)
  Rate Transition1/1 -> PPS EGO State Display/2(RPM)
  Data Type Conversion/1 -> Logical Operator4/2
  Pedestrian detection/9(ALARM) -> Rate Transition/1
  Logical Operator4/1 -> Terminator_1/1

== system NewModuleTry_cs/Audi_A8_1/ENABLED/PathFollower_1 ==
  TrajOffset_x,y,Y [m,m,deg] : Inport
  ActorOffset_Left(+) / Right(-) [m] : Inport  Port=2
  position x,y,Y [m,m,deg] : Inport  Port=3
  Initial Velocity [m/s] : Inport  Port=4
  Desired Velocity [m/s] : Inport  Port=5
  velocity [m/s] : Inport  Port=6
  CTRL REFERENCES : Subsystem
  Calculate shifted p0 wrt COG : Subsystem
  DELTA CTRL : Subsystem
  Demux : Demux  Outputs=3
  Gain : Gain  Gain=1*pi/180
  Goto Tag Visibility : GotoTagVisibility  GotoTag=PreviewDistance
  Goto Tag Visibility1 : GotoTagVisibility  GotoTag=v_actual
  Memory1 : Memory
  Memory2 : Memory
  Memory3 : Memory
  Mux : Mux  Inputs=3
  Preview distance  velocity dependent : Lookup  InputValues=[0 20 30 40 50 60 70 80 90 100 120]  Table=[1 1 2 3 4 5 6 7 10 13.33 20]
  THROTTLE CTRL : Subsystem
  sign1 : Gain  Gain=3.6
  delta_steerwheel [deg] : Outport
  throttle [%] : Outport  Port=2
  brake pressure [bar] : Outport  Port=3
  v0 [m/s] : Outport  Port=4
  Auto_GearShift : Outport  Port=5
  Actor/Traj_distance [m] : Outport  Port=6
  Actor/Traj_angle [deg] : Outport  Port=7
  tag scope: PreviewDistance=scoped, v_actual=scoped
  wires:
  Memory3/1 -> CTRL REFERENCES/4(ActorOffset_Left(+) / Right(-)_[m])
  THROTTLE CTRL/4(Auto_GearShift) -> Auto_GearShift/1
  THROTTLE CTRL/2(brake pressure [bar]) -> brake pressure [bar]/1
  Memory2/1 -> THROTTLE CTRL/1(v_actual [m/s]), [v_actual]
  Memory1/1 -> DELTA CTRL/1(p0), CTRL REFERENCES/1(Pos x,y,Y [m,m,rad])
  sign1/1 -> Preview distance  velocity dependent/1
  Initial Velocity [m/s]/1 -> THROTTLE CTRL/3(Initial Velocity [m/s])
  velocity [m/s]/1 -> Memory2/1
  CTRL REFERENCES/1(pvp  [m,m]) -> DELTA CTRL/2(pvp)
  CTRL REFERENCES/2(pref_pvp [m,m]) -> DELTA CTRL/3(pref_pvp)
  Gain/1 -> Mux/3
  DELTA CTRL/1(delta_steerwheel [deg]) -> delta_steerwheel [deg]/1
  Mux/1 -> CTRL REFERENCES/3(TrajOffset [m,m,rad])
  CTRL REFERENCES/3(pref_0 [m,m]) -> DELTA CTRL/4(pref0)
  THROTTLE CTRL/3(v0 [m/s]) -> v0 [m/s]/1
  THROTTLE CTRL/1(throttle [%]) -> throttle [%]/1
  [v_actual] -> sign1/1
  Preview distance  velocity dependent/1 -> [PreviewDistance], CTRL REFERENCES/2(Position Preview Distance [m])
  Desired Velocity [m/s]/1 -> THROTTLE CTRL/2(Desired Velocity [m/s])
  ActorOffset_Left(+) / Right(-) [m]/1 -> Memory3/1
  Demux/1 -> Mux/1
  Demux/2 -> Mux/2
  Demux/3 -> Gain/1
  TrajOffset_x,y,Y [m,m,deg]/1 -> Demux/1
  Calculate shifted p0 wrt COG/1(position x,y,Y [m,m,rad]) -> Memory1/1
  position x,y,Y [m,m,deg]/1 -> Calculate shifted p0 wrt COG/1(position x,y,Y [m,m,deg])
  CTRL REFERENCES/4(Actor/Traj_distance [m]) -> Actor/Traj_distance [m]/1
  CTRL REFERENCES/5(Actor/Traj_angle [deg]) -> Actor/Traj_angle [deg]/1

== system NewModuleTry_cs/Audi_A8_1/ENABLED/SELF_Demux ==
  SELF : Inport  OutDataTypeStr=Bus: PRESCAN_SELFSENSORDATA
  Bus Selector : BusSelector  OutputSignals=PositionX,PositionY,PositionZ,OrientationRoll,OrientationPitch,OrientationYaw,Velocity,Yaw_rate,Lat,Long,Alt
  Demux2 : Demux  Outputs=3
  Gain : Gain  Gain=180/pi
  Gain1 : Gain  Gain=180/pi
  Vector Concatenate1 : Concatenate  NumInputs=3
  compas converter : Subsystem
  x [m] : Outport
  y [m] : Outport  Port=2
  z [m] : Outport  Port=3
  rotx [deg] : Outport  Port=4
  roty [deg] : Outport  Port=5
  rotz [deg] : Outport  Port=6
  GPS lat [deg] : Outport  Port=7
  GPS long [deg] : Outport  Port=8
  GPS alt [m] : Outport  Port=9
  velocity [m/s] : Outport  Port=10
  heading [deg] : Outport  Port=11
  yaw rate [deg/s] : Outport  Port=12
  wires:
  Bus Selector/11 -> GPS alt [m]/1  "<Alt>"
  Bus Selector/10 -> GPS long [deg]/1  "<Long>"
  Bus Selector/9 -> GPS lat [deg]/1  "<Lat>"
  Bus Selector/8 -> Gain1/1  "<Yaw_rate>"
  Bus Selector/7 -> velocity [m/s]/1  "<Velocity>"
  Bus Selector/6 -> compas converter/1(rotz [rad]), Vector Concatenate1/3  "<OrientationYaw>"
  Bus Selector/5 -> Vector Concatenate1/2  "<OrientationPitch>"
  Bus Selector/4 -> Vector Concatenate1/1  "<OrientationRoll>"
  Vector Concatenate1/1 -> Gain/1
  Bus Selector/3 -> z [m]/1  "<PositionZ>"
  Bus Selector/2 -> y [m]/1  "<PositionY>"
  Bus Selector/1 -> x [m]/1  "<PositionX>"
  SELF/1 -> Bus Selector/1
  Gain/1 -> Demux2/1
  Demux2/1 -> rotx [deg]/1
  Demux2/2 -> roty [deg]/1
  Demux2/3 -> rotz [deg]/1
  compas converter/1(heading [deg]) -> heading [deg]/1
  Gain1/1 -> yaw rate [deg/s]/1

== system NewModuleTry_cs/Audi_A8_1/ENABLED/STATE_Audi_A8_1 ==
  State : Inport  SampleTime=TimeStep
  Bus Creator : BusCreator  Inputs=15  OutDataTypeStr=Bus: PRESCAN_STATEACTUATORDATA  NonVirtualBus=on
  Demux : Demux  Outputs=15
  iniBODYAngles wrtVEH [rad] : Constant  Value=[Roll0 Pitch0 0]  SampleTime=TimeStep
  iniVEHAngles wrtGLOB [rad] : Constant  Value=[0 0 Yaw0]  SampleTime=TimeStep
  iniVEHposition wrtGLOB [m] : Constant  Value=[x0 y0 z0]  SampleTime=TimeStep
  state2FullState : PreScanSimulinkLibrary/state2FullState  SystemSampleTime=-1
  StateBus : Outport  OutDataTypeStr=Bus: PRESCAN_STATEACTUATORDATA
  wires:
  Bus Creator/1 -> StateBus/1
  State/1 -> state2FullState/1
  state2FullState/1 -> Demux/1
  iniVEHposition wrtGLOB [m]/1 -> state2FullState/2
  iniBODYAngles wrtVEH [rad]/1 -> state2FullState/3
  iniVEHAngles wrtGLOB [rad]/1 -> state2FullState/4
  Demux/1 -> Bus Creator/1  "PositionX"
  Demux/2 -> Bus Creator/2  "PositionY"
  Demux/3 -> Bus Creator/3  "PositionZ"
  Demux/4 -> Bus Creator/4  "VelocityX"
  Demux/5 -> Bus Creator/5  "VelocityY"
  Demux/6 -> Bus Creator/6  "VelocityZ"
  Demux/7 -> Bus Creator/7  "AccelerationX"
  Demux/8 -> Bus Creator/8  "AccelerationY"
  Demux/9 -> Bus Creator/9  "AccelerationZ"
  Demux/10 -> Bus Creator/10  "OrientationRoll"
  Demux/11 -> Bus Creator/11  "OrientationPitch"
  Demux/12 -> Bus Creator/12  "OrientationYaw"
  Demux/13 -> Bus Creator/13  "AngularVelocityRoll"
  Demux/14 -> Bus Creator/14  "AngularVelocityPitch"
  Demux/15 -> Bus Creator/15  "AngularVelocityYaw"

== system NewModuleTry_cs/Audi_A8_1/ENABLED/State2PathFollowerCnv ==
  State BUS : Inport  OutDataTypeStr=Bus: PRESCAN_STATEACTUATORDATA
  Bus Selector : BusSelector  OutputSignals=AngularVelocityYaw,VelocityX,VelocityY,PositionX,PositionY,OrientationYaw
  Radians to Degrees : simulink_extras/Transformations/Radians to Degrees
  Radians to Degrees1 : simulink_extras/Transformations/Radians to Degrees
  SELF2PathFollowerMux : Mux  Tag=SELF2PathFollowerMux  Inputs=3
  velocity magnitude : Math  Operator=hypot  SaturateOnIntegerOverflow=on
  Yaw rate [deg/s] : Outport
  velocity [m/s] : Outport  Port=2
  position x,y,Y [m,m,deg] : Outport  Port=3
  wires:
  Radians to Degrees1/1 -> Yaw rate [deg/s]/1
  Bus Selector/1 -> Radians to Degrees1/1  "<AngularVelocityYaw>"
  velocity magnitude/1 -> velocity [m/s]/1
  SELF2PathFollowerMux/1 -> position x,y,Y [m,m,deg]/1
  State BUS/1 -> Bus Selector/1
  Bus Selector/2 -> velocity magnitude/1  "<VelocityX>"
  Bus Selector/3 -> velocity magnitude/2  "<VelocityY>"
  Radians to Degrees/1 -> SELF2PathFollowerMux/3
  Bus Selector/6 -> Radians to Degrees/1  "<OrientationYaw>"
  Bus Selector/4 -> SELF2PathFollowerMux/1  "<PositionX>"
  Bus Selector/5 -> SELF2PathFollowerMux/2  "<PositionY>"

== system NewModuleTry_cs/Audi_A8_1/ENABLED/TIS_2_StandardCoh_Demux ==
  TIS : Inport
  Bus Creator : BusCreator  Inputs=16
  Bus Selector : BusSelector  OutputSignals=ActiveBeamID[-],Range[m],DopplerVelocity[ms-1],DopplerVelocityX[ms-1],DopplerVelocityY[ms-1],DopplerVelocityZ[ms-1],Theta[deg],Phi[deg],TargetID[-],TargetTypeID[-],DopplerVelocityTranslationX[ms-1],DopplerVelocityTranslationY[ms-1],DopplerVelocityTranslationZ[ms-1],DopplerVelocityRotationX[ms-1],DopplerVelocityRotationY[ms-1],DopplerVelocityRotationZ[ms-1]
  ScannerSensorLegacyBusConversion : PreScanUsefulBlocks/ScannerSensorLegacyBusConversion  MAXMESSAGES=MAXMESSAGES
  Out1 : Outport
  Out2 : Outport  Port=2
  Out3 : Outport  Port=3
  Out4 : Outport  Port=4
  Out5 : Outport  Port=5
  Out7 : Outport  Port=6
  Out6 : Outport  Port=7
  wires:
  Bus Selector/16 -> Bus Creator/16  "<DopplerVelocityRotationZ[ms-1]>"
  Bus Selector/15 -> Bus Creator/15  "<DopplerVelocityRotationY[ms-1]>"
  Bus Selector/14 -> Bus Creator/14  "<DopplerVelocityRotationX[ms-1]>"
  Bus Selector/13 -> Bus Creator/13  "<DopplerVelocityTranslationZ[ms-1]>"
  Bus Selector/12 -> Bus Creator/12  "<DopplerVelocityTranslationY[ms-1]>"
  Bus Selector/11 -> Bus Creator/11  "<DopplerVelocityTranslationX[ms-1]>"
  ScannerSensorLegacyBusConversion/1 -> Bus Selector/1
  TIS/1 -> ScannerSensorLegacyBusConversion/1
  Bus Creator/1 -> Out6/1
  Bus Selector/10 -> Bus Creator/10  "<TargetTypeID[-]>"
  Bus Selector/9 -> Out7/1, Bus Creator/9  "<TargetID[-]>"
  Bus Selector/1 -> Out1/1, Bus Creator/1  "<ActiveBeamID[-]>"
  Bus Selector/2 -> Out2/1, Bus Creator/2  "<Range[m]>"
  Bus Selector/7 -> Out4/1, Bus Creator/7  "<Theta[deg]>"
  Bus Selector/8 -> Bus Creator/8, Out5/1  "<Phi[deg]>"
  Bus Selector/3 -> Bus Creator/3, Out3/1  "<DopplerVelocity[ms-1]>"
  Bus Selector/4 -> Bus Creator/4  "<DopplerVelocityX[ms-1]>"
  Bus Selector/5 -> Bus Creator/5  "<DopplerVelocityY[ms-1]>"
  Bus Selector/6 -> Bus Creator/6  "<DopplerVelocityZ[ms-1]>"
